simulink model "T_Junction_Lights"  (R2021a)
settings: Solver=VariableStepAuto  StartTime=0.0  StopTime=10.0  RelTol=1e-3
libraries: EdgesLibrary x21, StreetLanesLibrary x18
settings Model: Creator=timyb  LastModifiedBy=mariekutscher

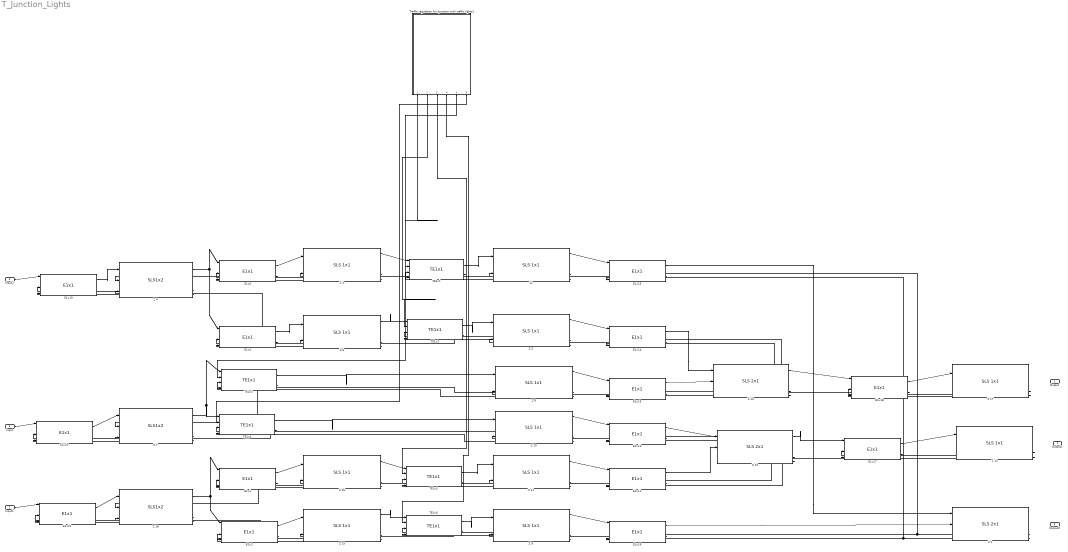
== system T_Junction_Lights ==
  Input : Inport
  Input1 : Inport  Port=2
  Input2 : Inport  Port=3
   Z {8..11,13,15..17} (8 alike) : StreetLanesLibrary/SLS 1x1  Kz=0  Tz=0
  " Z 3 " : StreetLanesLibrary/SLS 1x1  Kz=0  Tz=0
  E1x{1..2,5..6,11..21} (15 alike) : EdgesLibrary/E1x1
  TE1x{1..6} (6 alike) : EdgesLibrary/TE1x1  Rk=0
  Traffic regulation for tjunction with traffic lights1 : Stateflow chart  TreatAsAtomicUnit=on
  "Z 1 " : StreetLanesLibrary/SLS 2x1  Kz=0  Tz=0
  Z 12 : StreetLanesLibrary/SLS 2x1  Kz=0  Tz=0
  Z 14 : StreetLanesLibrary/SLS 2x1  Kz=0  Tz=0
  Z 18 : StreetLanesLibrary/SLS1x2  Kz=0  Tz=0
  Z 4 : StreetLanesLibrary/SLS1x2  Kz=0  Tz=0
  "Z 5 " : StreetLanesLibrary/SLS 1x1  Kz=0  Tz=0
  "Z 6 " : StreetLanesLibrary/SLS 1x1  Kz=0  Tz=0
  Z 7 : StreetLanesLibrary/SLS1x2  Kz=0  Tz=0
  "Z2 " : StreetLanesLibrary/SLS 1x1  Kz=0  Tz=0
  Output : Outport
  Output1 : Outport  Port=2
  Output2 : Outport  Port=3
  wires:
  E1x6/2 -> Z 4/2
  Z 4/2 -> E1x6/1, E1x5/1
  E1x5/2 -> Z 4/3
  E1x5/1 -> "Z 6 "/1
  "Z 6 "/8 -> E1x5/4
  "Z 6 "/7 -> E1x5/3
  E1x6/1 -> " Z 3 "/1
  " Z 3 "/8 -> E1x6/4
  " Z 3 "/7 -> E1x6/3
  "Z 6 "/2 -> TE1x2/1
  "Z 5 "/8 -> TE1x2/4
  "Z 5 "/7 -> TE1x2/3
  Z 7/2 -> TE1x3/1, TE1x4/1
  " Z 10"/7 -> TE1x4/3
  " Z 10"/8 -> TE1x4/4
  " Z 8"/8 -> TE1x3/4
  " Z 8"/7 -> TE1x3/3
  " Z 16"/2 -> TE1x5/1
  E1x1/2 -> Z 18/2
  Z 18/2 -> E1x2/1, E1x1/1
  E1x2/2 -> Z 18/3
  E1x2/1 -> " Z 15"/1
  " Z 15"/8 -> E1x2/4
  " Z 15"/7 -> E1x2/3
  E1x1/1 -> " Z 16"/1
  " Z 16"/8 -> E1x1/4
  " Z 16"/7 -> E1x1/3
  " Z 15"/2 -> TE1x6/1
  " Z 9"/8 -> TE1x6/4
  " Z 9"/7 -> TE1x6/3
  " Z 11"/8 -> TE1x5/4
  " Z 11"/7 -> TE1x5/3
  E1x16/2 -> " Z 9"/2
  " Z 9"/2 -> E1x16/1
  E1x16/1 -> "Z 1 "/2
  E1x15/1 -> "Z 1 "/1
  "Z 1 "/8 -> E1x15/4, E1x16/4
  "Z 1 "/7 -> E1x16/3, E1x15/3
  E1x17/1 -> " Z 13"/1
  " Z 13"/8 -> E1x17/4
  " Z 13"/7 -> E1x17/3
  E1x17/2 -> Z 12/3
  Z 12/2 -> E1x17/1
  E1x11/1 -> Z 12/2
  Z 12/8 -> E1x12/4, E1x11/4
  Z 12/7 -> E1x12/3, E1x11/3
  E1x12/1 -> Z 12/1
  E1x11/2 -> " Z 11"/2
  " Z 11"/2 -> E1x11/1
  E1x12/2 -> " Z 10"/2
  " Z 10"/2 -> E1x12/1
  E1x13/2 -> " Z 8"/2
  " Z 8"/2 -> E1x13/1
  E1x14/2 -> "Z 5 "/2
  "Z 5 "/2 -> E1x14/1
  E1x13/1 -> Z 14/2
  E1x14/1 -> Z 14/1
  Z 14/8 -> E1x14/4, E1x13/4
  Z 14/7 -> E1x14/3, E1x13/3
  E1x18/2 -> Z 14/3
  Z 14/2 -> E1x18/1
  E1x18/1 -> " Z 17"/1
  " Z 17"/8 -> E1x18/4
  " Z 17"/7 -> E1x18/3
  E1x15/2 -> "Z2 "/2
  "Z2 "/2 -> E1x15/1
  Z 4/7 -> E1x19/3
  E1x19/1 -> Z 4/1
  Z 4/8 -> E1x19/4
  Input2/1 -> E1x19/1
  E1x20/1 -> Z 7/1
  Z 7/8 -> E1x20/4
  Z 7/7 -> E1x20/3
  Input/1 -> E1x20/1
  Input1/1 -> E1x21/1
  Z 18/7 -> E1x21/3
  Z 18/8 -> E1x21/4
  E1x21/1 -> Z 18/1
  " Z 3 "/2 -> TE1x1/1
  "Z2 "/7 -> TE1x1/3
  "Z2 "/8 -> TE1x1/4
  TE1x1/2 -> " Z 3 "/2
  TE1x1/1 -> "Z2 "/1
  TE1x2/2 -> "Z 6 "/2
  TE1x2/1 -> "Z 5 "/1
  TE1x3/1 -> " Z 8"/1
  TE1x3/2 -> Z 7/2
  TE1x4/1 -> " Z 10"/1
  TE1x4/2 -> Z 7/3
  TE1x5/2 -> " Z 16"/2
  TE1x5/1 -> " Z 11"/1
  TE1x6/1 -> " Z 9"/1
  TE1x6/2 -> " Z 15"/2
  Traffic regulation for tjunction with traffic lights1/1(enable1) -> TE1x1/2
  Traffic regulation for tjunction with traffic lights1/2(enable2) -> TE1x2/2
  Traffic regulation for tjunction with traffic lights1/4(enable4) -> TE1x6/2
  Traffic regulation for tjunction with traffic lights1/3(enable3) -> TE1x5/2
  Traffic regulation for tjunction with traffic lights1/6(enable6) -> TE1x4/2
  Traffic regulation for tjunction with traffic lights1/5(enable5) -> TE1x3/2

== stateflow chart T_Junction_Lights/Traffic regulation for tjunction with traffic lights1 ==
  state Lane1_3_5
    entry: counter = 0;
    enable1 = true;
    enable3 = true;
    enable5 = true;
    counter = counter + 1;
    exit: enable1 = false; enable3 = false; enable5 = false;
  state Lane1_2_3
    entry: counter = 0;
    enable1 = true;
    enable2 = true;
    enable3 = true;
    counter = counter + 1;
    exit: enable1 = false; enable2 = false; enable3 = false;
  state Lane3_4_5
    entry: counter = 0;
    enable3 = true;
    enable4 = true;
    enable5 = true;
    counter = counter + 1;
    exit: enable3 = false; enable4 = false; enable5 = false;
  state Lane1_6
    entry: counter=0;
    enable1 = true;
    enable6 = true;
    counter = counter + 1;
    exit: enable1 = false; enable6 = false;
  (default) -> Lane1_3_5
  Lane1_6 -> Lane1_3_5 : [counter > 5]
  Lane1_3_5 -> Lane1_2_3 : [counter > 5]
  Lane1_2_3 -> Lane3_4_5 : [counter > 5]
  Lane3_4_5 -> Lane1_6 : [counter > 5]
  data: enable1 output boolean size=1; enable2 output boolean size=1; enable3 output boolean size=1; enable4 output boolean size=1; enable5 output boolean size=1; enable6 output boolean size=1; l5 local; l6 local; counter local; l1 local; l2 local; l4 local; l3 local
